simulink model "lab8_model_nonlinear"  (R2022a)
settings: Solver=FixedStepAuto  StartTime=0.0  StopTime=300  FixedStep=0.001  RelTol=1e-3
values from neighbouring files (symbols this model uses):
  A = pi*2.25^2    (= 15.9043128088)    [Lab8.m]    (also in linear_workspace.mat; nonlinear_workspace.mat)
  c1 = 6.7767    [Lab8.m]    (also in linear_workspace.mat; nonlinear_workspace.mat)
  c2 = 6.5198    [Lab8.m]    (also in linear_workspace.mat; nonlinear_workspace.mat)
  Kd = (2*zeta*omega + alpha - b2) / b1    [Lab8.m]    (also in linear_workspace.mat = 34.2521231491; nonlinear_workspace.mat = 34.2521231491)
  Ki = (alpha*omega^2) / b1    [Lab8.m]    (also in linear_workspace.mat = 0.514641540244; nonlinear_workspace.mat = 0.514641540244)
  km = 3.614    [Lab8.m]    (also in linear_workspace.mat; nonlinear_workspace.mat)
  Kp = (omega^2 + 2*alpha*zeta*omega - b3) / b1    [Lab8.m]    (also in linear_workspace.mat = 4.56614097638; nonlinear_workspace.mat = 4.56614097638)
settings Model: Creator=ahmcmillon  LastModifiedBy=ahmcmillon
settings DataIOCC: ReturnWorkspaceOutputs=off

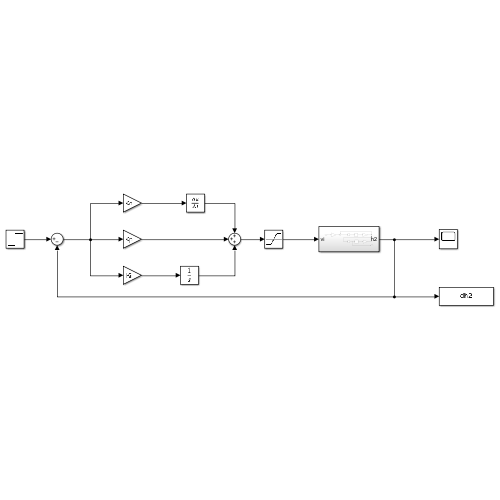
[thumbnail: Simulink's stored preview of the top-level diagram]
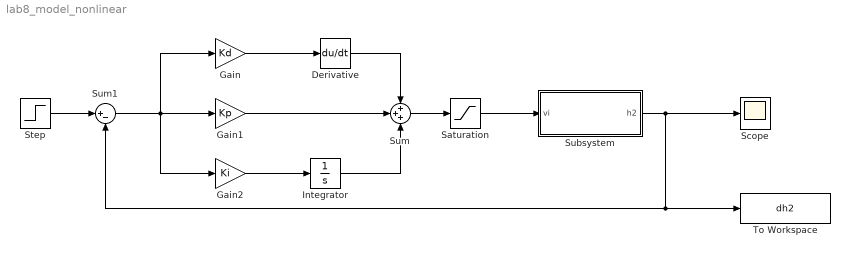
== system lab8_model_nonlinear ==
  Derivative : Derivative
  Gain : Gain  Gain=Kd
  Gain1 : Gain  Gain=Kp
  Gain2 : Gain  Gain=Ki
  Integrator : Integrator
  Saturation : Saturate  UpperLimit=22  LowerLimit=0
  Scope : Scope
  Step : Step  Time=150  Before=10  After=12  SampleTime=0
  Subsystem : Subsystem
  Sum : Sum  Inputs=+++
  Sum1 : Sum  Inputs=|+-
  To Workspace : ToWorkspace  VariableName=dh2  SaveFormat=Structure With Time  SampleTime=-1
  wires:
  Step/1 -> Sum1/1
  Sum1/1 -> Gain2/1, Gain/1, Gain1/1
  Gain2/1 -> Integrator/1
  Gain1/1 -> Sum/2
  Integrator/1 -> Sum/3
  Gain/1 -> Derivative/1
  Derivative/1 -> Sum/1
  Subsystem/1(h2) -> Sum1/2, To Workspace/1, Scope/1
  Sum/1 -> Saturation/1
  Saturation/1 -> Subsystem/1(vi)

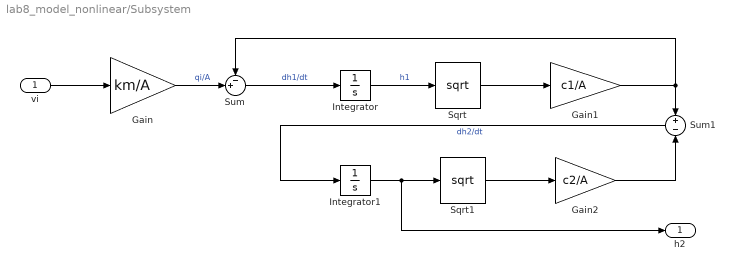
== system lab8_model_nonlinear/Subsystem ==
  vi : Inport
  Gain : Gain  Gain=km/A
  Gain1 : Gain  Gain=c1/A
  Gain2 : Gain  Gain=c2/A
  Integrator : Integrator
  Integrator1 : Integrator
  Sqrt : Sqrt
  Sqrt1 : Sqrt
  Sum : Sum  Inputs=-+|
  Sum1 : Sum  Inputs=+-
  h2 : Outport
  wires:
  vi/1 -> Gain/1
  Gain/1 -> Sum/2  "qi/A"
  Sum/1 -> Integrator/1  "dh1/dt"
  Gain1/1 -> Sum1/1, Sum/1
  Gain2/1 -> Sum1/2
  Sum1/1 -> Integrator1/1  "dh2/dt"
  Integrator1/1 -> h2/1, Sqrt1/1
  Integrator/1 -> Sqrt/1  "h1"
  Sqrt/1 -> Gain1/1
  Sqrt1/1 -> Gain2/1
